simulink model "fuzzyControllerTestBench"  (R2013b)
settings: Solver=FixedStepDiscrete  StartTime=0.0  StopTime=1  RelTol=1e-3
libraries: fuzblock x1
settings Model: NumberOfSteps=10  Creator=Raj  LastModifiedBy=Raj
settings OptimizationCC: UseIntDivNetSlope=on  UseFloatMulNetSlope=on  OptimizeModelRefInitCode=on  LifeSpan=1  MaxStackSize=64
settings HardwareCC: ProdLargestAtomicInteger=Long  ProdLargestAtomicFloat=Double  ProdIntDivRoundTo=Zero  ProdEndianess=LittleEndian  ProdHWDeviceType=ARM Compatible->ARM Cortex
settings RTWCC: SystemTargetFile=ert.tlc  GenCodeOnly=on  TemplateMakefile=ert_default_tmf  Description=Embedded Coder  ProcessScript=ert_make_rtw_hook  Toolchain=GNU Tools for ARM Embedded Processors
settings CodeAppCC: IgnoreCustomStorageClasses=off
settings ERTTargetCC: CodeReplacementLibrary=ANSI_C  IncludeMdlTerminateFcn=off  SuppressErrorStatus=on  SupportNonFinite=off  ERTCustomFileTemplate=example_file_process.tlc  ConvertIfToSwitch=on

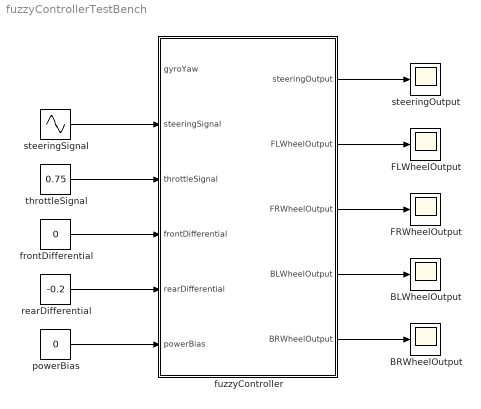
== system fuzzyControllerTestBench ==
  BLWheelOutput : Scope
      settings: SaveName=ScopeData3
  BRWheelOutput : Scope
      settings: SaveName=ScopeData4
  FLWheelOutput : Scope
  FRWheelOutput : Scope
      settings: SaveName=ScopeData2
  frontDifferential : Constant  Value=0
  fuzzyController : Subsystem
  powerBias : Constant  Value=0
  rearDifferential : Constant  Value=-0.2
  steeringOutput : Scope
  steeringSignal : Sin  Frequency=5  SampleTime=0
  throttleSignal : Constant  Value=0.75
  wires:
  throttleSignal/1 -> fuzzyController/3(throttleSignal)
  frontDifferential/1 -> fuzzyController/4(frontDifferential)
  rearDifferential/1 -> fuzzyController/5(rearDifferential)
  powerBias/1 -> fuzzyController/6(powerBias)
  fuzzyController/1(steeringOutput) -> steeringOutput/1
  fuzzyController/2(FLWheelOutput) -> FLWheelOutput/1
  fuzzyController/3(FRWheelOutput) -> FRWheelOutput/1
  fuzzyController/4(BLWheelOutput) -> BLWheelOutput/1
  fuzzyController/5(BRWheelOutput) -> BRWheelOutput/1
  steeringSignal/1 -> fuzzyController/2(steeringSignal)

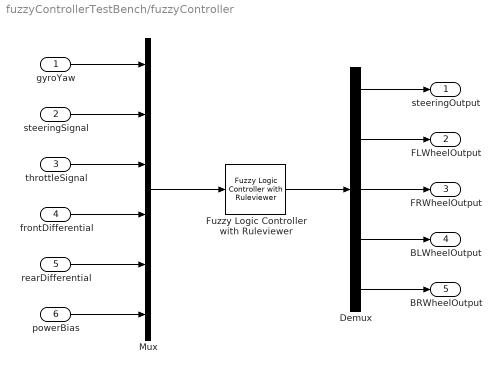
== system fuzzyControllerTestBench/fuzzyController ==
  gyroYaw : Inport
  steeringSignal : Inport  Port=2
  throttleSignal : Inport  Port=3
  frontDifferential : Inport  Port=4
  rearDifferential : Inport  Port=5
  powerBias : Inport  Port=6
  Demux : Demux  Outputs=5
  Fuzzy Logic Controller with Ruleviewer : fuzblock/Fuzzy Logic  Controller  with Ruleviewer  fismatrix=fuzzyController  Ts=0.01
  Mux : Mux  Inputs=6
  steeringOutput : Outport
  FLWheelOutput : Outport  Port=2
  FRWheelOutput : Outport  Port=3
  BLWheelOutput : Outport  Port=4
  BRWheelOutput : Outport  Port=5
  wires:
  gyroYaw/1 -> Mux/1
  steeringSignal/1 -> Mux/2
  frontDifferential/1 -> Mux/4
  Fuzzy Logic Controller with Ruleviewer/1 -> Demux/1
  powerBias/1 -> Mux/6
  Demux/4 -> BLWheelOutput/1
  Demux/3 -> FRWheelOutput/1
  Demux/1 -> steeringOutput/1
  Mux/1 -> Fuzzy Logic Controller with Ruleviewer/1
  Demux/2 -> FLWheelOutput/1
  Demux/5 -> BRWheelOutput/1
  rearDifferential/1 -> Mux/5
  throttleSignal/1 -> Mux/3
